simulink library "otter_controllers"  (R2024a)
settings: Solver=VariableStepAuto  StartTime=0.0  StopTime=10.0  RelTol=1e-3
undefined symbols (not defined in the file or in its folder): data, db_params, deepc_params, params
libraries: $bdroot x3, sim_lib x1, data_driven_lib_ctl x1, mpclib x1, slpidlib x1
settings Model: Creator=mandicluka  LastModifiedBy=luka
settings RTWCC: GPUComputeCapability=3.5

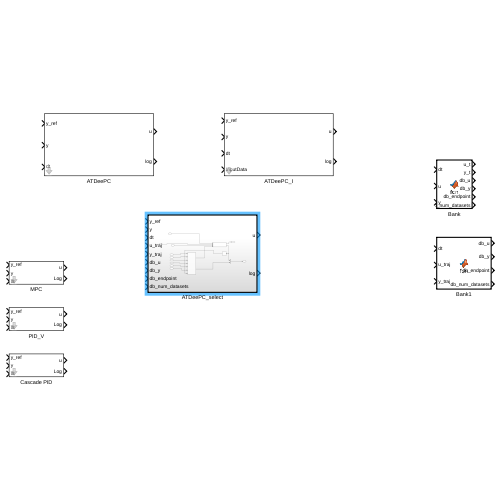
[thumbnail: Simulink's stored preview of the top-level diagram]
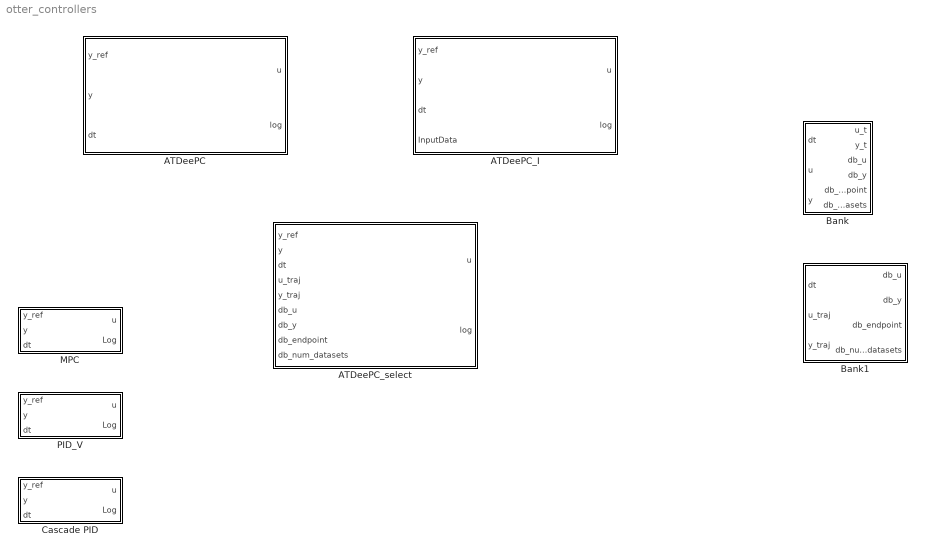
== system otter_controllers ==
  ATDeePC : Subsystem  Tag=controller;  mask{params=deepc_params, trajectory_T=0, data=0, db_params=0, linearization_n=2}
      mask prompts: params "Parameter struct:"
  ATDeePC_I : Subsystem  Tag=controller;  mask{params=deepc_params, trajectory_T=0, data=0, db_params=0}
      mask prompts: params "Parameter struct:"
  ATDeePC_select : Subsystem  TreatAsAtomicUnit=on
  Bank : MATLAB Function  TreatAsAtomicUnit=on
  Bank1 : MATLAB Function  TreatAsAtomicUnit=on
  Cascade PID : Subsystem  mask{params=params}
      mask prompts: params "Param Struct:"
  MPC : Subsystem  mask{params=0}
      mask prompts: params "MPC params"
  PID_V : Subsystem  mask{params=params.params_v}
      mask prompts: params "Param Struct:"

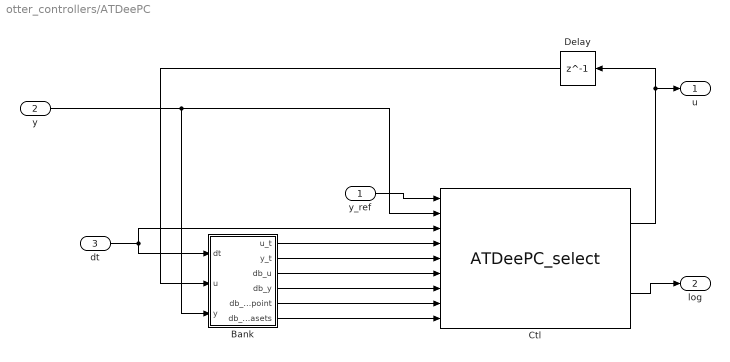
== system otter_controllers/ATDeePC ==
  y_ref : Inport
  y : Inport  Port=2
  dt : Inport  Port=3
  Bank : MATLAB Function  TreatAsAtomicUnit=on
  Ctl : $bdroot/ATDeePC_select  SystemSampleTime=-1  VariantActivationTime=update diagram  AllowFlexibleInterface=on  Latency=0  AutoFrameSizeCalculation=off
      link override ATDeePC1: params=params.deepc_params
  Delay : Delay  DelayLength=1
  u : Outport
  log : Outport  Port=2
  wires:
  y/1 -> Bank/3(y), Ctl/2
  y_ref/1 -> Ctl/1
  dt/1 -> Bank/1(dt), Ctl/3
  Ctl/1 -> Delay/1, u/1
  Ctl/2 -> log/1
  Delay/1 -> Bank/2(u)
  Bank/1(u_t) -> Ctl/4
  Bank/2(y_t) -> Ctl/5
  Bank/3(db_u) -> Ctl/6
  Bank/4(db_y) -> Ctl/7
  Bank/5(db_endpoint) -> Ctl/8
  Bank/6(db_num_datasets) -> Ctl/9

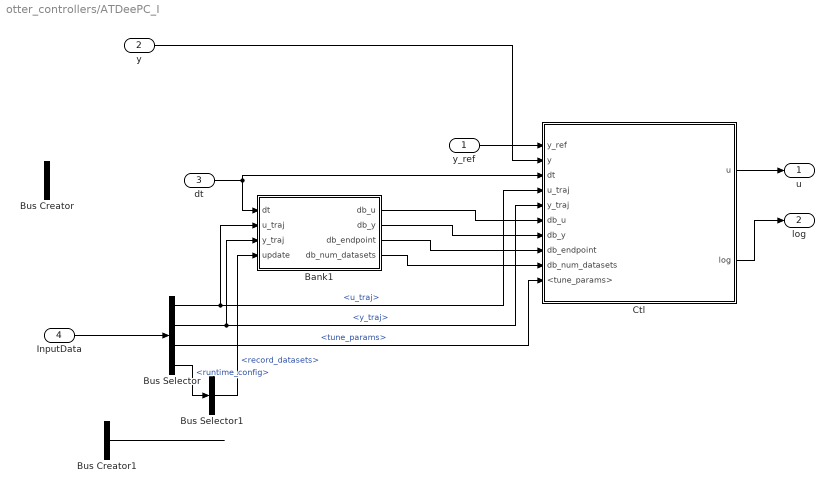
== system otter_controllers/ATDeePC_I ==
  y_ref : Inport
  y : Inport  Port=2
  dt : Inport  Port=3
  InputData : Inport  Port=4
  Bank1 : MATLAB Function  TreatAsAtomicUnit=on
  Bus Creator : BusCreator  Inputs=4
  Bus Creator1 : BusCreator  Inputs=1
  Bus Selector : BusSelector  OutputSignals=u_traj,y_traj,tune_params,runtime_config
  Bus Selector1 : BusSelector  OutputSignals=record_datasets
  Ctl : Subsystem  TreatAsAtomicUnit=on
  u : Outport
  log : Outport  Port=2
  wires:
  y/1 -> Ctl/2(y)
  y_ref/1 -> Ctl/1(y_ref)
  dt/1 -> Bank1/1(dt), Ctl/3(dt)
  Ctl/1(u) -> u/1
  Ctl/2(log) -> log/1
  Bus Selector/1 -> Bank1/2(u_traj), Ctl/4(u_traj)  "<u_traj>"
  Bank1/1(db_u) -> Ctl/6(db_u)
  Bank1/2(db_y) -> Ctl/7(db_y)
  Bank1/3(db_endpoint) -> Ctl/8(db_endpoint)
  Bank1/4(db_num_datasets) -> Ctl/9(db_num_datasets)
  Bus Selector/2 -> Bank1/3(y_traj), Ctl/5(y_traj)  "<y_traj>"
  ? -> Bus Creator/1  "u_traj"
  ? -> Bus Creator/2  "y_traj"
  ? -> Bus Creator/3  "tune_params"
  Bus Selector/3 -> Ctl/10(<tune_params>)  "<tune_params>"
  ? -> Bus Creator/4  "runtime_config"
  InputData/1 -> Bus Selector/1
  Bus Selector/4 -> Bus Selector1/1  "<runtime_config>"
  Bus Selector1/1 -> Bank1/4(update)  "<record_datasets>"
  ? -> Bus Creator1/1  "record_datasets"
  Bus Creator1/1 -> ?

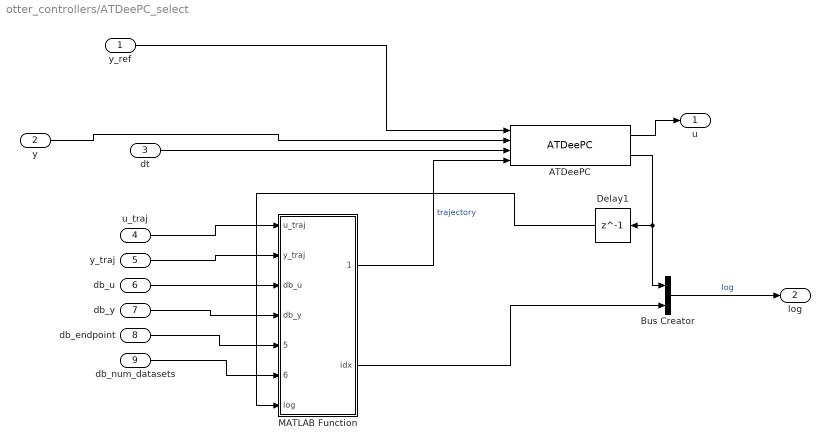
== system otter_controllers/ATDeePC_select ==
  y_ref : Inport
  y : Inport  Port=2
  dt : Inport  Port=3
  u_traj : Inport  Port=4
  y_traj : Inport  Port=5
  db_u : Inport  Port=6
  db_y : Inport  Port=7
  db_endpoint : Inport  Port=8
  db_num_datasets : Inport  Port=9
  ATDeePC : data_driven_lib_ctl/ATDeePC  Tag=__cs_comptype:ctl;__cs_compimpl:mat;  iid__=[0]  pid__=[65 84 68 101 101 80 67 58 100 97 116 97 95 100 114 105 118 101 110 95 108 105 98]  params=params.deepc_params  LogEntryType=ATDeePC_LT  data=ATDeePC_data  ParamsType=ATDeePC_PT  DataType=ATDeePC_DT  u_ic=0  trajectory_T=ATDeePC_trajectory_T
  Bus Creator : BusCreator  Inputs=2
  Delay1 : Delay  DelayLength=1
  MATLAB Function : MATLAB Function  TreatAsAtomicUnit=on
  u : Outport
  log : Outport  Port=2
  wires:
  y/1 -> ATDeePC/2
  y_ref/1 -> ATDeePC/1
  dt/1 -> ATDeePC/3
  ATDeePC/1 -> u/1
  ATDeePC/2 -> Bus Creator/1, Delay1/1
  MATLAB Function/1(trajectory) -> ATDeePC/4  "trajectory"
  Delay1/1 -> MATLAB Function/7(log)
  u_traj/1 -> MATLAB Function/1(u_traj)
  y_traj/1 -> MATLAB Function/2(y_traj)
  Bus Creator/1 -> log/1  "log"
  MATLAB Function/2(idx) -> Bus Creator/2
  db_u/1 -> MATLAB Function/3(db_u)
  db_y/1 -> MATLAB Function/4(db_y)
  db_endpoint/1 -> MATLAB Function/5(db_static_gain)
  db_num_datasets/1 -> MATLAB Function/6(db_num_datasets)

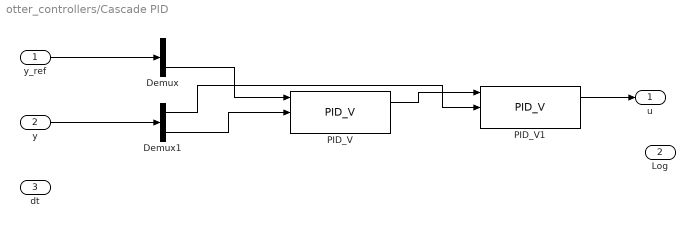
== system otter_controllers/Cascade PID ==
  y_ref : Inport
  y : Inport  Port=2
  dt : Inport  Port=3
  Demux : Demux  Outputs=2
  Demux1 : Demux  Outputs=2
  PID_V : $bdroot/PID_V  params=params.params_p
  PID_V1 : $bdroot/PID_V  params=params.params_v
  u : Outport
  Log : Outport  Port=2
  wires:
  y_ref/1 -> Demux/1
  y/1 -> Demux1/1
  Demux/2 -> PID_V/1
  Demux1/2 -> PID_V/2
  PID_V/1 -> PID_V1/1
  PID_V1/1 -> u/1
  Demux1/1 -> PID_V1/2

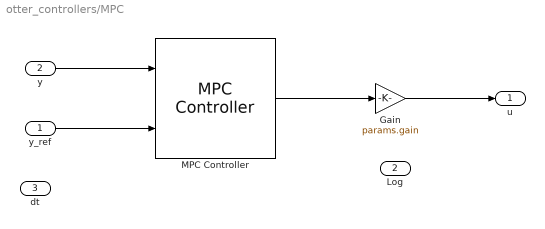
== system otter_controllers/MPC ==
  y_ref : Inport
  y : Inport  Port=2
  dt : Inport  Port=3
  Gain : Gain  Gain=params.gain
  MPC Controller : mpclib/MPC Controller  SCDEnableBlockLinearizationSpecification=on  mpcobj=params.mpc  is_multiple=0  enable_value=0  return_u0=off  updateMPCinCallerWorkspace=on  md_inport=off  mv_inport=off  uref_inport=off  return_cost=off  return_mvseq=off  return_qpstatus=off  return_xseq=off  return_state=off  return_ovseq=off  state_inport=off  umin_inport=off  umax_inport=off  ymin_inport=off  ymax_inport=off  cc_inport=off  ywt_inport=off  uwt_inport=off  duwt_inport=off  rhoeps_inport=off  pm_inport=off  MaximumP=10  HorizonChoice=FixedHorizon  n_ts=1  n_p=10  n_mv=1  n_md=1  n_ud=0  n_mo=1  n_uo=0  BlockDataType=double  SampleTimeInherited=off  switch_inport=off
  u : Outport
  Log : Outport  Port=2
  wires:
  MPC Controller/1 -> Gain/1
  y_ref/1 -> MPC Controller/2
  y/1 -> MPC Controller/1
  Gain/1 -> u/1

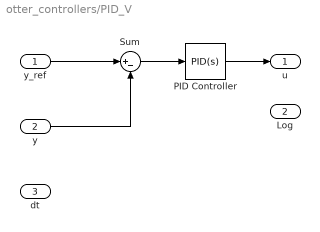
== system otter_controllers/PID_V ==
  y_ref : Inport
  y : Inport  Port=2
  dt : Inport  Port=3
  PID Controller : slpidlib/PID Controller  Controller=PID  Form=Parallel  TimeDomain=Continuous-time  UseExternalTs=off  SampleTime=-1  IntegratorMethod=Forward Euler  FilterMethod=Forward Euler  ControllerParametersSource=internal  P=params.K_p  I=params.K_i  UseKiTs=off  D=params.K_d  UseExternalDerivativeSource=off  N=params.K_N  UseFilter=on  TunerSelectOption=Transfer Function Based (PID Tuner App)  InitialConditionSource=internal  InitialConditionForIntegrator=0  InitialConditionForFilter=0  DifferentiatorICPrevScaledInput=0  ExternalReset=none  TrackingMode=off  Kt=1  LimitOutput=on  SatLimitsSource=internal  UpperSaturationLimit=params.saturation.max  LowerSaturationLimit=params.saturation.min  LinearizeAsGain=on  AntiWindupMode=clamping  Kb=1  LimitIntegrator=off  UpperIntegratorSaturationLimit=inf  LowerIntegratorSaturationLimit=-inf  POutMin=[]  POutMax=[]  IOutMin=[]  IOutMax=[]  DOutMin=[]  DOutMax=[]  NOutMin=[]  NOutMax=[]  SumOutMin=[]  SumOutMax=[]  SaturationOutMin=[]  SaturationOutMax=[]  PParamMin=[]  PParamMax=[]  IParamMin=[]  IParamMax=[]  DParamMin=[]  DParamMax=[]  NParamMin=[]  NParamMax=[]  KbParamMin=[]  KbParamMax=[]  KtParamMin=[]  KtParamMax=[]  KbOutMin=[]  KbOutMax=[]  KtOutMin=[]  KtOutMax=[]  IntegratorOutMin=[]  IntegratorOutMax=[]  FilterOutMin=[]  FilterOutMax=[]  SumI1OutMin=[]  SumI1OutMax=[]  SumI2OutMin=[]  SumI2OutMax=[]  SumI3OutMin=[]  SumI3OutMax=[]  SumI4OutMin=[]  SumI4OutMax=[]  SumDOutMin=[]  SumDOutMax=[]  DifferentiatorOutMin=[]  DifferentiatorOutMax=[]  FilterDiffOutCoefMin=[]  FilterDiffOutCoefMax=[]  ReciprocalOutMin=[]  ReciprocalOutMax=[]  SumDenOutMin=[]  SumDenOutMax=[]  SumNumOutMin=[]  SumNumOutMax=[]  DivideOutMin=[]  DivideOutMax=[]  UdiffTsProdOutMin=[]  UdiffTsProdOutMax=[]  NTsProdOutMin=[]  NTsProdOutMax=[]  UintegralTsProdOutMin=[]  UintegralTsProdOutMax=[]  UngainTsProdOutMin=[]  UngainTsProdOutMax=[]  ClampingZeroOutDataTypeStr=Inherit: Inherit via back propagation  ClampingZeroOutMin=[]  ClampingZeroOutMax=[]  FilterDenConstantOutDataTypeStr=Inherit: Inherit via back propagation  FilterDenConstantOutMin=[]  FilterDenConstantOutMax=[]  PCopyOutDataTypeStr=Inherit: Inherit via back propagation  PCopyOutMin=[]  PCopyOutMax=[]  NCopyOutDataTypeStr=Inherit: Inherit via back propagation  NCopyOutMin=[]  NCopyOutMax=[]  IntegratorContinuousStateAttributes=''  IntegratorStateMustResolveToSignalObject=off  IntegratorRTWStateStorageClass=Auto  FilterContinuousStateAttributes=''  FilterStateMustResolveToSignalObject=off  FilterRTWStateStorageClass=Auto  ParallelPVariant=InternalParameters  IdealPVariant=Disabled  IVariant=InternalParameters  DVariant=InternalParameters  IntegratorVariant=Continuous  SatVariant=Enabled  AWVariant=ContClampingParallel  PCopyVariant=Disabled  TRVariant=Disabled  FdbkBlocksVariant=Forward  IdealPFdbkVariant=Disabled  SatFdbkVariant=Disabled  DerivativeFilterVariant=ContFilter  NVariant=InternalParameters  NCopyVariant=Disabled  FilterICVariant=InternalICsFilter  IntegratorICVariant=InternalICs  ExternalResetVariant=Disabled  TRSumVariant=Passthrough  SumFdbkVariant=Disabled  SumVariant=Sum_PID  TsampFilterVariant=InternalTs  TsampNgainVariant=Passthrough  TsampIntegralVariant=Disabled_SignalSpec  ExternalSaturationOutDataTypeStr=Inherit: Same as second input  DerivativeSourceVariant=ErrorSignal
  Sum : Sum  Inputs=|+-
  u : Outport
  Log : Outport  Port=2
  wires:
  Sum/1 -> PID Controller/1
  y/1 -> Sum/2
  y_ref/1 -> Sum/1
  PID Controller/1 -> u/1

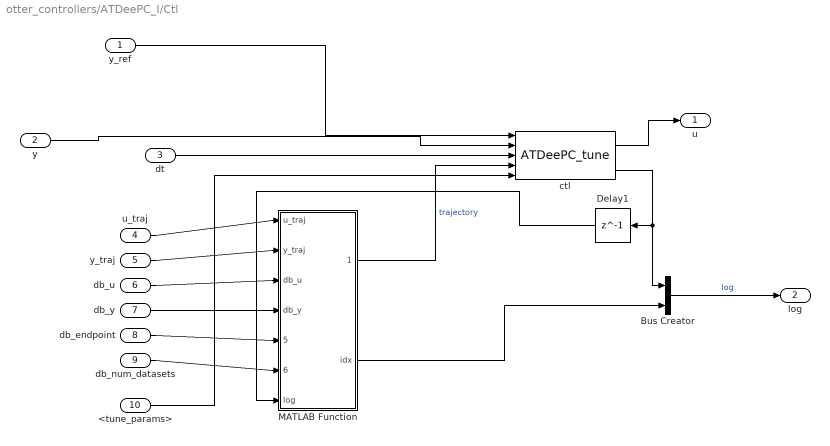
== system otter_controllers/ATDeePC_I/Ctl ==
  y_ref : Inport
  y : Inport  Port=2
  dt : Inport  Port=3
  u_traj : Inport  Port=4
  y_traj : Inport  Port=5
  db_u : Inport  Port=6
  db_y : Inport  Port=7
  db_endpoint : Inport  Port=8
  db_num_datasets : Inport  Port=9
  <tune_params> : Inport  Port=10
  Bus Creator : BusCreator  Inputs=2
  Delay1 : Delay  DelayLength=1
  MATLAB Function : MATLAB Function  TreatAsAtomicUnit=on
  ctl : sim_lib/Controllers/ATDeePC_tune  Tag=controller;m_controller;  params=params.deepc_params  data=atdeepc_tune_data  LogEntryType=ATDeePC_tune_LT  ParamsType=ATDeePC_tune_PT  DataType=ATDeePC_tune_DT  trajectory_T=ATDeePC_tune_trajectory_T  tune_params_T=ATDeePC_tune_tune_params_T
  u : Outport
  log : Outport  Port=2
  wires:
  db_num_datasets/1 -> MATLAB Function/6(db_num_datasets)
  db_endpoint/1 -> MATLAB Function/5(db_endpoint)
  db_y/1 -> MATLAB Function/4(db_y)
  db_u/1 -> MATLAB Function/3(db_u)
  MATLAB Function/2(idx) -> Bus Creator/2
  Bus Creator/1 -> log/1  "log"
  y_traj/1 -> MATLAB Function/2(y_traj)
  u_traj/1 -> MATLAB Function/1(u_traj)
  Delay1/1 -> MATLAB Function/7(log)
  MATLAB Function/1(trajectory) -> ctl/4  "trajectory"
  ctl/2 -> Delay1/1, Bus Creator/1
  ctl/1 -> u/1
  dt/1 -> ctl/3
  y_ref/1 -> ctl/1
  y/1 -> ctl/2
  <tune_params>/1 -> ctl/5

== matlab function otter_controllers/ATDeePC/Bank ==
  settings: updateMethod=DISCRETE
  data: u_t output; y_t output; dt input; db_u output; u input; y input; db_params parameter; data parameter; db_y output; db_endpoint output; db_num_datasets output
function [u_t, y_t, db_u, db_y, db_endpoint, db_num_datasets] = fcn(dt, u, y, db_params, data)

    persistent t u_traj y_traj last_changed_t db_u_p db_y_p db_endpoint_p db_num_datasets_p    

    traj_len = data.T;
    if isempty(t)
        t = 0;
        last_changed_t = 0;
        db_num_datasets_p = db_params.num_datasets_in_bank;
        db_u_p = zeros(db_params.dataset_bank_size, data.T, data.m);
        db_y_p = zeros(db_params.dataset_bank_size, data.T, data.p);
        db_endpoint_p = zeros(db_params.dataset_bank_size, data.m);
        if db_num_datasets_p > 0
            db_u_p(end-db_num_datasets_p+1, :, :) = db_params.D_u;
            db_y_p(end-db_num_datasets_p+1, :, :) = db_params.D_y;
            db_endpoint_p(end-db_num_datasets_p+1, :, :) = db_params.end_point;
        end
        u_traj = zeros(traj_len, data.m);
        y_traj = zeros(traj_len, data.p);
    end

    t = t + dt;

    coder.extrinsic('trajectory_dataset'); % arx function not supported
    u_traj = circshift(u_traj, -1);
    y_traj = circshift(y_traj, -1);
    u_traj(end, :) = u(db_params.input_record_dims);
    y_traj(end, :) = y(db_params.output_record_dims);

    u_t = u_traj;
    y_t = y_traj;    
    
    
    [t, last_changed_t, db_u_p, db_y_p, db_endpoint_p, db_num_datasets_p, ...
       db_u, db_y, db_endpoint, db_num_datasets] = ...
          update_dataset_bank(t, last_changed_t, db_u_p, db_y_p, db_endpoint_p, db_num_datasets_p, dt, u_traj, y_traj, db_params, data);

end

== matlab function otter_controllers/ATDeePC_select/MATLAB Function ==
  settings: updateMethod=DISCRETE
  data: u_traj input; y_traj input; db_u input; db_y input; db_static_gain input; db_num_datasets input; trajectory output trajectory_T; log input; db_params parameter; data parameter; idx output
function [trajectory, idx] = fcn(u_traj, y_traj, db_u, db_y, db_static_gain, db_num_datasets, log, db_params, data)

    persistent last_n_ds trajectory_p i

    if isempty(last_n_ds)
        last_n_ds = 1;
        i = last_n_ds;
        trajectory_p = struct( ...
            'D_u', zeros(data.T, data.m), ...
            'D_y', zeros(data.T, data.p), ...
            'static_gain', zeros(data.m, 1));
        trajectory_p.D_u(:, :) = db_u(end-i+1, :, :);
        trajectory_p.D_y(:, :) = db_y(end-i+1, :, :);
        trajectory_p.static_gain(:) = db_static_gain(end-i+1, :);
        trajectory = trajectory_p;
        idx = i;
        return
    end

    if db_params.dataset_mode == 0
        trajectory = trajectory_p;
        idx = i;
        return
    end

    if db_params.dataset_mode == 1
        if db_num_datasets > last_n_ds
            i = db_num_datasets;
            trajectory_p.D_u(:, :) = db_u(end-i+1, :, :);
            trajectory_p.D_y(:, :) = db_y(end-i+1, :, :);
            trajectory_p.static_gain(:) = db_static_gain(end-i+1, :);
            last_n_ds = db_num_datasets;
        end
        trajectory = trajectory_p;
        idx = i;
        return
    end
    
    if db_params.traj_mode == 2
        [u_t, y_t] = compose_trajectory_with_prediction(u_traj, y_traj, log.x_op_u, log.x_op_y);
    else
        u_t = u_traj;
        y_t = y_traj;
    end

    i = select_current_datasets(db_u, db_y, db_num_datasets, i, u_t, y_t, db_params);
    trajectory_p.D_u(:, :) = db_u(end-i+1, :, :);
    trajectory_p.D_y(:, :) = db_y(end-i+1, :, :);
    trajectory_p.static_gain(:) = db_static_gain(end-i+1, :);

    trajectory = trajectory_p;
    idx = i;

end

== matlab function otter_controllers/Bank ==
  settings: updateMethod=DISCRETE
  data: u_t output; y_t output; dt input; db_u output; u input; y input; db_params parameter; data parameter; db_y output; db_endpoint output; db_num_datasets output
function [u_t, y_t, db_u, db_y, db_endpoint, db_num_datasets] = fcn(dt, u, y, db_params, data)

    persistent t u_traj y_traj last_changed_t db_u_p db_y_p db_endpoint_p db_num_datasets_p    

    traj_len = data.T;
    if isempty(t)
        u_traj = zeros(traj_len, data.m);
        y_traj = zeros(traj_len, data.p);
        t = 0;
        db_num_datasets_p = db_params.num_datasets_in_bank;
        db_u_p = zeros(db_params.dataset_bank_size, data.m, data.T);
        db_y_p = zeros(db_params.dataset_bank_size, data.p, data.T);
        db_endpoint_p = zeros(db_params.dataset_bank_size, data.m);
        if db_num_datasets_p > 0
            db_u_p(end-db_num_datasets_p+1, :, :) = db_params.D_u;
            db_y_p(end-db_num_datasets_p+1, :, :) = db_params.D_y;
            db_endpoint_p(end-db_num_datasets_p+1, :, :) = db_params.end_point;
        end
        last_changed_t = 0;
    end

    t = t + dt;

    coder.extrinsic('trajectory_dataset'); % arx function not supported
    u_traj = circshift(u_traj, -1);
    y_traj = circshift(y_traj, -1);
    u_traj(end, :) = u(db_params.input_record_dims);
    y_traj(end, :) = y(db_params.output_record_dims);

    u_t = u_traj;
    y_t = y_traj;    
    
    
    [t, last_changed_t, db_u_p, db_y_p, db_endpoint_p, db_num_datasets_p, ...
       db_u, db_y, db_endpoint, db_num_datasets] = ...
          update_dataset_bank(t, last_changed_t, db_u_p, db_y_p, db_endpoint_p, db_num_datasets_p, dt, u_traj, y_traj, db_params, data);

end

== matlab function otter_controllers/Bank1 ==
  settings: updateMethod=DISCRETE
  data: dt input; db_u output; u_traj input; y_traj input; db_params parameter; data parameter; db_y output; db_endpoint output; db_num_datasets output
function [db_u, db_y, db_endpoint, db_num_datasets] = fcn(dt, u_traj, y_traj, db_params, data)

    persistent t last_changed_t db_u_p db_y_p db_endpoint_p db_num_datasets_p
    
    if isempty(t)
        t = 0;
        db_num_datasets_p = db_params.num_datasets_in_bank;
        db_u_p = zeros(db_params.dataset_bank_size, data.m, data.T);
        db_y_p = zeros(db_params.dataset_bank_size, data.p, data.T);
        db_endpoint_p = zeros(db_params.dataset_bank_size, data.m);
        if db_num_datasets_p > 0
            db_u_p(end-db_num_datasets_p+1, :, :) = db_params.D_u;
            db_y_p(end-db_num_datasets_p+1, :, :) = db_params.D_y;
            db_endpoint_p(end-db_num_datasets_p+1, :, :) = db_params.end_point;
        end
        last_changed_t = 0;
    end
    
    [t, last_changed_t, db_u_p, db_y_p, db_endpoint_p, db_num_datasets_p, ...
       db_u, db_y, db_endpoint, db_num_datasets] = ...
          update_dataset_bank(t, last_changed_t, db_u_p, db_y_p, db_endpoint_p, db_num_datasets_p, dt, u_traj, y_traj, db_params, data);


end

== matlab function otter_controllers/ATDeePC_I/Bank1 ==
  settings: updateMethod=DISCRETE
  data: dt input; db_u output; u_traj input; y_traj input; update input; db_params parameter; data parameter; db_y output; db_endpoint output; db_num_datasets output
function [db_u, db_y, db_endpoint, db_num_datasets] = fcn(dt, u_traj, y_traj, update, db_params, data)

    persistent t last_changed_t db_u_p db_y_p db_endpoint_p db_num_datasets_p
    
    if isempty(t)
        t = 0;
        db_num_datasets_p = db_params.num_datasets_in_bank;
        db_u_p = zeros(db_params.dataset_bank_size, data.m, data.T);
        db_y_p = zeros(db_params.dataset_bank_size, data.p, data.T);
        db_endpoint_p = zeros(db_params.dataset_bank_size, data.m);
        if db_num_datasets_p > 0
            db_u_p(end-db_num_datasets_p+1, :, :) = db_params.D_u;
            db_y_p(end-db_num_datasets_p+1, :, :) = db_params.D_y;
            db_endpoint_p(end-db_num_datasets_p+1, :, :) = db_params.end_point;
        end
        last_changed_t = 0;
    end

    if update <= 0
        db_u = db_u_p;
        db_y = db_y_p;
        db_endpoint = db_endpoint_p;
        db_num_datasets = db_num_datasets_p;
        return
    end
    
    [t, last_changed_t, db_u_p, db_y_p, db_endpoint_p, db_num_datasets_p, ...
       db_u, db_y, db_endpoint, db_num_datasets] = ...
          update_dataset_bank(t, last_changed_t, db_u_p, db_y_p, db_endpoint_p, db_num_datasets_p, dt, u_traj, y_traj, db_params, data);


end

== matlab function otter_controllers/ATDeePC_I/Ctl/MATLAB Function ==
  settings: updateMethod=DISCRETE
  data: u_traj input; y_traj input; db_u input; db_y input; db_endpoint input; db_num_datasets input; trajectory output trajectory_T; log input; db_params parameter; data parameter; idx output
function [trajectory, idx] = fcn(u_traj, y_traj, db_u, db_y, db_endpoint, db_num_datasets, log, db_params, data)

    persistent last_n_ds trajectory_p i

    if isempty(last_n_ds)
        last_n_ds = 1;
        i = last_n_ds;
        trajectory_p = struct( ...
            'D_u', zeros(data.m, data.T), ...
            'D_y', zeros(data.p, data.T), ...
            'end_point', zeros(data.m));
        trajectory_p.D_u(:, :) = db_u(end-i+1, :, :);
        trajectory_p.D_y(:, :) = db_y(end-i+1, :, :);
        trajectory_p.end_point(:) = db_endpoint(end-i+1, :);
        trajectory = trajectory_p;
        idx = i;
        return
    end

    if db_params.dataset_mode == 0
        trajectory = trajectory_p;
        idx = i;
        return
    end

    if db_params.dataset_mode == 1
        if db_num_datasets > last_n_ds
            i = db_num_datasets;
            trajectory_p.D_u(:, :) = db_u(end-i+1, :, :);
            trajectory_p.D_y(:, :) = db_y(end-i+1, :, :);
            trajectory_p.end_point(:) = db_endpoint(end-i+1, :);
            last_n_ds = db_num_datasets;
        end
        trajectory = trajectory_p;
        idx = i;
        return
    end

    [u_t, y_t] = compose_trajectory_with_prediction(u_traj, y_traj, log.x_op_u, log.x_op_y, db_params.traj_mode);
    i = select_current_datasets(db_u, db_y, db_num_datasets, i, u_t, y_t, db_params);
    trajectory_p.D_u(:, :) = db_u(end-i+1, :, :);
    trajectory_p.D_y(:, :) = db_y(end-i+1, :, :);
    trajectory = trajectory_p;
    idx = i;

end
